simulink model "main_gilbert"  (R2023a)
settings: Solver=VariableStepAuto  StartTime=0.0  StopTime=3  FixedStep=0.01  RelTol=1e-3
libraries: commchan3 x2, dspvision x2, commrandsrc3 x1
settings Model: Creator=avyamalhotra  LastModifiedBy=mitul
settings OptimizationCC: ReuseModelBlockBuffer=off

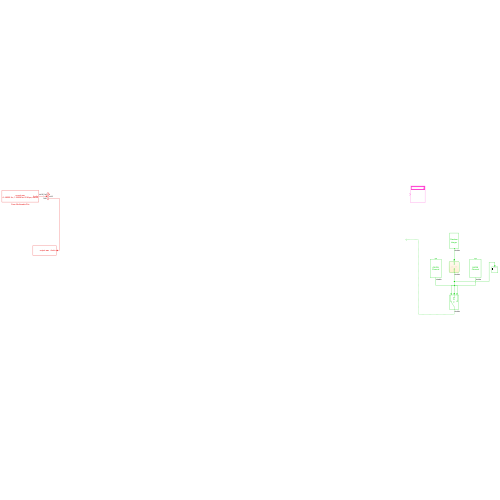
[thumbnail: Simulink's stored preview of the top-level diagram]
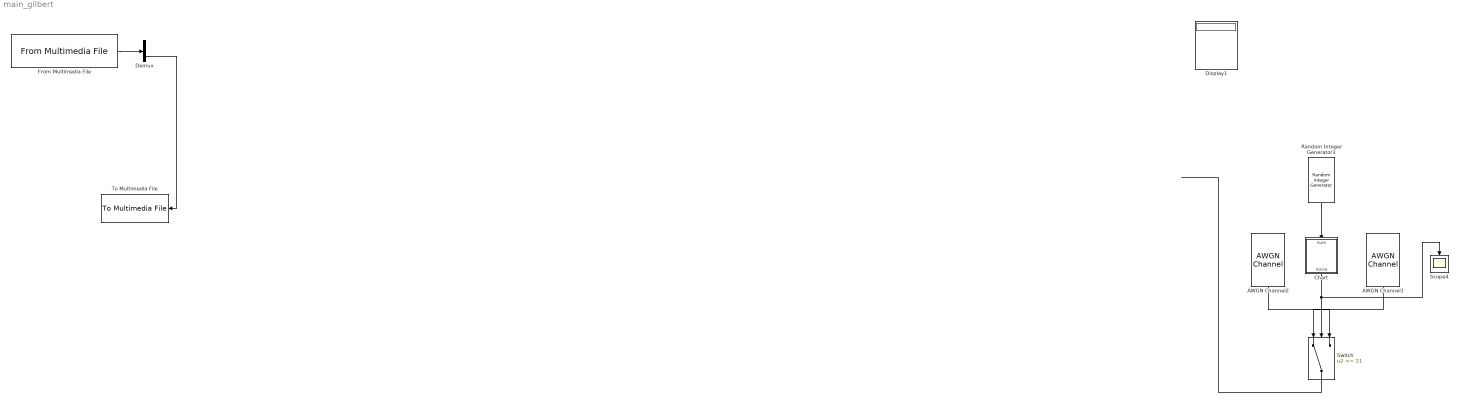
== system main_gilbert ==
  AWGN Channel1 : commchan3/AWGN Channel  LegacyMode=on  NoiseMethod="Signal to noise ratio  (SNR)"  noiseMode="Signal to noise ratio  (SNR)"  EbNo=2  EsNo=10  SNR=21  BitsPerSymbol=4  SignalPower=1  SamplesPerSymbol=1  SymbolPeriod=1  VarianceSource=Parameter  Variance=1  RandomStream=Global stream  Seed=67  SimulateUsing=Code generation
  AWGN Channel2 : commchan3/AWGN Channel  LegacyMode=on  NoiseMethod="Signal to noise ratio  (SNR)"  noiseMode="Signal to noise ratio  (SNR)"  EbNo=2  EsNo=10  SNR=9  BitsPerSymbol=4  SignalPower=1  SamplesPerSymbol=1  SymbolPeriod=1  VarianceSource=Parameter  Variance=1  RandomStream=Global stream  Seed=67  SimulateUsing=Code generation
  Chart : Stateflow chart  TreatAsAtomicUnit=on
  Demux : Demux  Outputs=2
  Display1 : Display
  From Multimedia File : dspvision/From Multimedia File  inputFilename=C:\Users\mitul\Downloads\sound.wav  readRange=[1 Inf]  loop=on  numPlays=1  outputStreams=Audio only  videoDataType=single  audioDataType=int16  inheritSampleTime=on  userDefinedSampleTime=1/30  noAudioOutput=off  isIntensityVideo=off  fourcc=RGB  colorVideoFormat=Separate color signals  outputEOF=off  dataOrg=Column-major  audioFrameSize=1  computeAudioFrameSize=off  outSamplingMode=Sample based
      settings: LibrarySourceBlock=dspsrcs4/From Multimedia File
  Random Integer Generator3 : commrandsrc3/Random Integer Generator  SetSize=101  SeedSource=Parameter  Seed=9  SampleTime=1e-4  SamplesPerFrame=1  OutputDataType=double  SimulateUsing=Interpreted execution
  Scope4 : Scope
  Switch : Switch  Threshold=21  SaturateOnIntegerOverflow=off  InputSameDT=off
  To Multimedia File : dspvision/To Multimedia File  outputFilename=C:\Users\mitul\Desktop\FPGAW2\output.wav  streamSelection=Audio only  videoCompressor=None (uncompressed)  audioCompressor=None (uncompressed)  imagePorts=Separate color signals  fileType=WAV  audioDatatype=16-bit integer  fourcc=RGB  videoQuality=75  mj2000CompFactor=10
      settings: LibrarySourceBlock=dspsnks4/To Multimedia File
  wires:
  From Multimedia File/1 -> Demux/1
  Switch/1 -> ?
  AWGN Channel2/1 -> Switch/3
  AWGN Channel1/1 -> Switch/1
  Random Integer Generator3/1 -> Chart/1(num)
  Chart/1(noise) -> Scope4/1, Switch/2
  Demux/2 -> To Multimedia File/1

== stateflow chart main_gilbert/Chart ==
  state Good_state
    noise=21;
  state Bad_state
    noise=9;
  (default) -> Good_state
  Bad_state -> Bad_state [order 2] : [num<=75]
  Good_state -> Bad_state [order 1] : [num<=3]
  Good_state -> Good_state [order 2] : [num<=97]
  Bad_state -> Good_state [order 1] : [num<=25]
  data: noise output; num input
